simulink model "sampleModel106"  (R2022a)
settings: Solver=VariableStepAuto  StartTime=0.0  StopTime=10.0  RelTol=1e-3
undefined symbols (not defined in the file): DiscIntNeverNeededParam, magnitude, Newton, Raphson
libraries: simulink x379, slpidlib x89
(part 5 of 16)

== system sampleModel106/cfblk82/cfblk7/cfblk7 ==
  cfblk1 : Inport
  cfblk14 : Inport  Port=2
  cfblk15 : Inport  Port=3
  cfblk16 : Inport  Port=4
  cfblk10 : Constant  Value=[138530855.287176]  SampleTime=1
  cfblk11 : Constant  Value=[847049310.105778]  SampleTime=1
  cfblk12 : Subsystem
  cfblk13 : Subsystem
  cfblk17 : Delay  SampleTime=1
  cfblk18 : Delay  SampleTime=1
  cfblk3 : DiscreteFilter  SampleTime=1
  cfblk4 : simulink/Discrete/Transfer Fcn Real Zero  ZeroZ=0.75  ICPrevInput=0.0  DoSatur=off
      settings: SourceProductBaseCode=SL
  cfblk5 : DiscreteTransferFcn  SampleTime=1
  cfblk6 : DiscreteFilter  SampleTime=1
  cfblk7 : Sum  Inputs=+-
  cfblk8 : Assignment  DiagnosticForDimensions=Warning  IndexOptions=Index vector (dialog)  Indices=1  OutputSizes=1
  cfblk9 : Abs  SaturateOnIntegerOverflow=off
  cfblk2 : Outport
  wires:
  cfblk3/1 -> cfblk8/1, cfblk7/2
  cfblk10/1 -> cfblk12/1(cfblk1)
  cfblk9/1 -> cfblk13/1(cfblk1)
  cfblk15/1 -> cfblk12/2(cfblk6)
  cfblk11/1 -> cfblk2/1
  cfblk16/1 -> cfblk9/1
  cfblk6/1 -> cfblk4/1
  cfblk4/1 -> cfblk3/1
  cfblk8/1 -> cfblk5/1
  cfblk5/1 -> cfblk12/3(cfblk7)
  cfblk14/1 -> cfblk12/4(cfblk8)
  cfblk1/1 -> cfblk13/3(cfblk14)
  cfblk13/1(cfblk2) -> cfblk7/1
  cfblk13/2(cfblk15) -> cfblk6/1, cfblk12/5(cfblk9)
  cfblk7/1 -> cfblk17/1
  cfblk17/1 -> cfblk13/2(cfblk13)
  cfblk12/1(cfblk2) -> cfblk18/1
  cfblk18/1 -> cfblk8/2

== system sampleModel106/cfblk82/cfblk7/cfblk8 ==
  cfblk1 : Inport
  cfblk15 : Inport  Port=2
  cfblk10 : Constant  Value=[796043451.416910]  SampleTime=1
  cfblk11 : Subsystem
  cfblk12 : Subsystem
  cfblk13 : Subsystem
  cfblk14 : If  IfExpression=u1 >= 0  SampleTime=1
  cfblk18 : Subsystem  TreatAsAtomicUnit=on
  cfblk19 : Subsystem  TreatAsAtomicUnit=on
  cfblk20 : Delay  SampleTime=1
  cfblk21 : Delay  SampleTime=1
  cfblk22 : Delay  SampleTime=1
  cfblk3 : DiscreteZeroPole  Poles=[0 0.5]  Gain=1
  cfblk4 : DiscreteTransferFcn  SampleTime=1
  cfblk5 : Signum
  cfblk6 : Sum  Inputs=-+
  cfblk7 : UnaryMinus
  cfblk8 : Signum
  cfblk9 : UnaryMinus
  cfblk2 : Outport
  cfblk16 : Outport  Port=2
  cfblk17 : Outport  Port=3
  wires:
  cfblk19/1(cfblk2) -> cfblk12/2(cfblk6)
  cfblk15/1 -> cfblk14/1
  cfblk3/1 -> cfblk11/1(cfblk1)
  cfblk13/1(cfblk2) -> cfblk2/1
  cfblk12/1(cfblk2) -> cfblk8/1
  cfblk12/2(cfblk7) -> cfblk9/1
  cfblk4/1 -> cfblk5/1
  cfblk1/1 -> cfblk19/1(cfblk1)
  cfblk19/2(cfblk7) -> cfblk6/1
  cfblk6/1 -> cfblk3/1
  cfblk8/1 -> cfblk6/2
  cfblk18/1(cfblk2) -> cfblk16/1
  cfblk5/1 -> cfblk13/1(cfblk1)
  cfblk12/3(cfblk8) -> cfblk13/2(cfblk14)
  cfblk11/1(cfblk2) -> cfblk7/1
  cfblk18/2(cfblk7) -> cfblk4/1
  cfblk10/1 -> cfblk13/3(cfblk15)
  cfblk11/2(cfblk11) -> cfblk17/1
  cfblk11/3(cfblk12) -> cfblk13/4(cfblk16)
  cfblk14/1 -> cfblk18/Action
  cfblk14/2 -> cfblk19/Action
  cfblk7/1 -> cfblk20/1
  cfblk20/1 -> cfblk12/1(cfblk1)
  cfblk13/2(cfblk17) -> cfblk21/1
  cfblk21/1 -> cfblk11/2(cfblk10)
  cfblk9/1 -> cfblk22/1
  cfblk22/1 -> cfblk18/1(cfblk1)

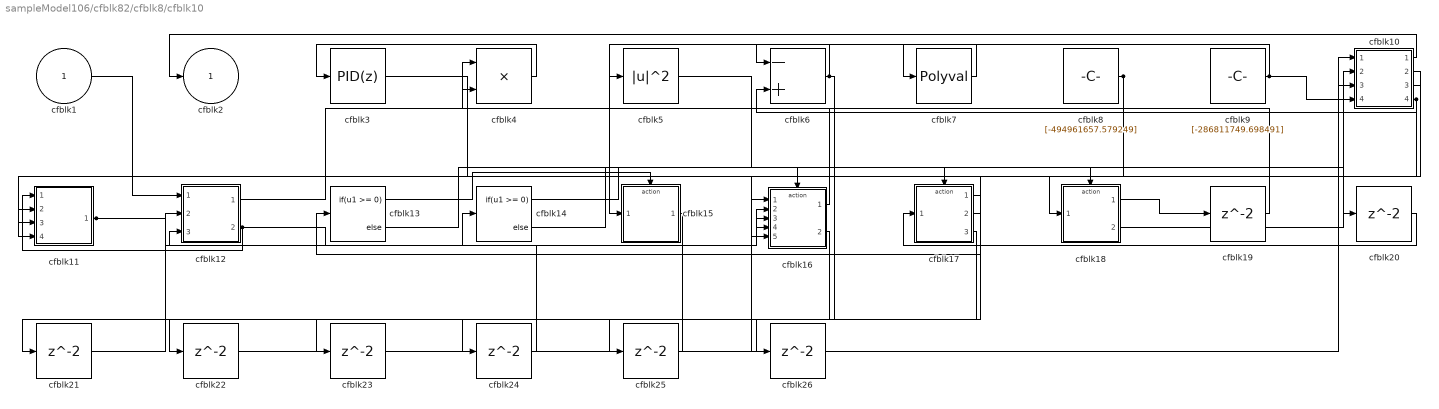
== system sampleModel106/cfblk82/cfblk8/cfblk10 ==
  cfblk1 : Inport
  cfblk10 : Subsystem
  cfblk11 : Subsystem
  cfblk12 : Subsystem
  cfblk13 : If  IfExpression=u1 >= 0  SampleTime=1
  cfblk14 : If  IfExpression=u1 >= 0  SampleTime=1
  cfblk15 : Subsystem  TreatAsAtomicUnit=on
  cfblk16 : Subsystem  TreatAsAtomicUnit=on
  cfblk17 : Subsystem  TreatAsAtomicUnit=on
  cfblk18 : Subsystem  TreatAsAtomicUnit=on
  cfblk{19..26} (8 alike) : Delay  SampleTime=1
  cfblk3 : slpidlib/PID Controller  Controller=PID  Form=Parallel  TimeDomain=Discrete-time  UseExternalTs=off  SampleTime=1  IntegratorMethod=Forward Euler  FilterMethod=Forward Euler  ControllerParametersSource=internal  P=1  I=1  UseKiTs=off  D=0  N=100  UseFilter=on  TunerSelectOption=Transfer Function Based (PID Tuner App)  InitialConditionSource=internal  InitialConditionForIntegrator=0  InitialConditionForFilter=0  DifferentiatorICPrevScaledInput=0  ExternalReset=none  TrackingMode=off  Kt=1  LimitOutput=off  SatLimitsSource=internal  UpperSaturationLimit=inf  LowerSaturationLimit=-inf  LinearizeAsGain=off  AntiWindupMode=none  Kb=1  POutMin=[]  POutMax=[]  IOutMin=[]  IOutMax=[]  DOutMin=[]  DOutMax=[]  NOutMin=[]  NOutMax=[]  SumOutMin=[]  SumOutMax=[]  SaturationOutMin=[]  SaturationOutMax=[]  PParamMin=[]  PParamMax=[]  IParamMin=[]  IParamMax=[]  DParamMin=[]  DParamMax=[]  NParamMin=[]  NParamMax=[]  KbParamMin=[]  KbParamMax=[]  KtParamMin=[]  KtParamMax=[]  KbOutMin=[]  KbOutMax=[]  KtOutMin=[]  KtOutMax=[]  IntegratorOutMin=[]  IntegratorOutMax=[]  FilterOutMin=[]  FilterOutMax=[]  SumI1OutMin=[]  SumI1OutMax=[]  SumI2OutMin=[]  SumI2OutMax=[]  SumI3OutMin=[]  SumI3OutMax=[]  SumI4OutMin=[]  SumI4OutMax=[]  SumDOutMin=[]  SumDOutMax=[]  DifferentiatorOutMin=[]  DifferentiatorOutMax=[]  FilterDiffOutCoefMin=[]  FilterDiffOutCoefMax=[]  ReciprocalOutMin=[]  ReciprocalOutMax=[]  SumDenOutMin=[]  SumDenOutMax=[]  SumNumOutMin=[]  SumNumOutMax=[]  DivideOutMin=[]  DivideOutMax=[]  UdiffTsProdOutMin=[]  UdiffTsProdOutMax=[]  NTsProdOutMin=[]  NTsProdOutMax=[]  UintegralTsProdOutMin=[]  UintegralTsProdOutMax=[]  UngainTsProdOutMin=[]  UngainTsProdOutMax=[]  IntegratorContinuousStateAttributes=''  IntegratorStateMustResolveToSignalObject=off  IntegratorRTWStateStorageClass=Auto  FilterContinuousStateAttributes=''  FilterStateMustResolveToSignalObject=off  FilterRTWStateStorageClass=Auto  ParallelPVariant=InternalParameters  IdealPVariant=Disabled  IVariant=InternalParameters  DVariant=InternalParameters  IntegratorVariant=Discrete  SatVariant=Disabled  AWVariant=Passthrough  PCopyVariant=Disabled  TRVariant=Disabled  FdbkBlocksVariant=Forward  IdealPFdbkVariant=Disabled  SatFdbkVariant=Disabled  DerivativeFilterVariant=ForwardEulerFilter  NVariant=InternalParameters  NCopyVariant=Disabled  FilterICVariant=InternalICsFilter  IntegratorICVariant=InternalICs  ExternalResetVariant=Disabled  TRSumVariant=Passthrough  SumFdbkVariant=Disabled  SumVariant=Sum_PID  TsampFilterVariant=InternalTs  TsampNgainVariant=Passthrough  TsampIntegralVariant=Passthrough  ExternalSaturationOutDataTypeStr=Inherit: Same as second input  aMode=0
  cfblk4 : Product
  cfblk5 : Math  Operator=magnitude^2
  cfblk6 : Sum  Inputs=-+
  cfblk7 : Polyval  Coefs=[ +2.081618890e-019, -1.441693666e-014, +4.719686976e-010, -8.536869453e-006, +1.621573104e-001, -8.087801117e+001 ]
  cfblk8 : Constant  Value=[-494961657.579249]  SampleTime=1
  cfblk9 : Constant  Value=[-286811749.698491]  SampleTime=1
  cfblk2 : Outport
  wires:
  cfblk1/1 -> cfblk12/1(cfblk1)
  cfblk9/1 -> cfblk7/1, cfblk10/4(cfblk12)
  cfblk8/1 -> cfblk13/1, cfblk16/5(cfblk15)
  cfblk4/1 -> cfblk3/1
  cfblk6/1 -> cfblk15/1(cfblk1), cfblk26/1
  cfblk7/1 -> cfblk6/1
  cfblk3/1 -> cfblk18/1(cfblk1)
  cfblk12/1(cfblk2) -> cfblk4/1
  cfblk12/2(cfblk11) -> cfblk11/1(cfblk1), cfblk16/4(cfblk14)
  cfblk10/1(cfblk2) -> cfblk2/1
  cfblk16/1(cfblk2) -> cfblk5/1
  cfblk11/1(cfblk2) -> cfblk16/2(cfblk12), cfblk16/3(cfblk13)
  cfblk10/2(cfblk13) -> cfblk11/2(cfblk11)
  cfblk18/2(cfblk13) -> cfblk10/2(cfblk10)
  cfblk10/3(cfblk14) -> cfblk11/3(cfblk12)
  cfblk10/4(cfblk15) -> cfblk6/2, cfblk11/4(cfblk13)
  cfblk13/1 -> cfblk15/Action
  cfblk13/2 -> cfblk16/Action
  cfblk14/1 -> cfblk17/Action
  cfblk14/2 -> cfblk18/Action
  cfblk18/1(cfblk2) -> cfblk19/1
  cfblk19/1 -> cfblk4/2
  cfblk5/1 -> cfblk20/1
  cfblk20/1 -> cfblk17/1(cfblk1)
  cfblk17/1(cfblk2) -> cfblk21/1
  cfblk21/1 -> cfblk12/2(cfblk9)
  cfblk17/2(cfblk10) -> cfblk22/1
  cfblk22/1 -> cfblk16/1(cfblk1)
  cfblk17/3(cfblk11) -> cfblk23/1
  cfblk23/1 -> cfblk10/1(cfblk1)
  cfblk16/2(cfblk16) -> cfblk24/1
  cfblk24/1 -> cfblk14/1
  cfblk15/1(cfblk2) -> cfblk25/1
  cfblk25/1 -> cfblk12/3(cfblk10)
  cfblk26/1 -> cfblk10/3(cfblk11)

== system sampleModel106/cfblk83/cfblk11/cfblk10 ==
  cfblk1 : Inport
  cfblk12 : Inport  Port=2
  cfblk10 : Constant  Value=[-915348538.475738]  SampleTime=1
  cfblk11 : If  IfExpression=u1 >= 0  SampleTime=1
  cfblk14 : Subsystem  TreatAsAtomicUnit=on
  cfblk15 : Subsystem  TreatAsAtomicUnit=on
  cfblk{16..20} (5 alike) : Delay  SampleTime=1
  cfblk3 : DiscreteIntegrator  ICPrevOutput=DiscIntNeverNeededParam  ICPrevScaledInput=DiscIntNeverNeededParam
  cfblk4 : simulink/Discrete/Transfer Fcn Lead or Lag  PoleZ=0.95  ZeroZ=0.75  ICPrevOutput=0.0  ICPrevInput=0.0  DoSatur=off
      settings: SourceProductBaseCode=SL
  cfblk5 : UnitDelay  HasFrameUpgradeWarning=on
  cfblk6 : Sum  Inputs=|++
  cfblk7 : Squeeze
  cfblk8 : Sum  Inputs=+-
  cfblk9 : Sum  Inputs=|++
  cfblk2 : Outport
  cfblk13 : Outport  Port=2
  wires:
  cfblk5/1 -> cfblk2/1, cfblk16/1
  cfblk3/1 -> cfblk7/1
  cfblk4/1 -> cfblk8/1
  cfblk12/1 -> cfblk14/1(cfblk1)
  cfblk14/1(cfblk2) -> cfblk15/2(cfblk13)
  cfblk9/1 -> cfblk4/1
  cfblk8/1 -> cfblk6/1, cfblk14/3(cfblk7)
  cfblk6/1 -> cfblk11/1
  cfblk15/1(cfblk2) -> cfblk5/1, cfblk3/1, cfblk18/1
  cfblk1/1 -> cfblk9/2
  cfblk10/1 -> cfblk14/2(cfblk6)
  cfblk14/3(cfblk10) -> cfblk13/1, cfblk15/3(cfblk14), cfblk20/1
  cfblk11/1 -> cfblk14/Action
  cfblk11/2 -> cfblk15/Action
  cfblk16/1 -> cfblk8/2
  cfblk7/1 -> cfblk17/1
  cfblk17/1 -> cfblk15/1(cfblk1)
  cfblk18/1 -> cfblk14/4(cfblk8)
  cfblk14/2(cfblk9) -> cfblk19/1
  cfblk19/1 -> cfblk9/1
  cfblk20/1 -> cfblk6/2

== system sampleModel106/cfblk83/cfblk11/cfblk11 ==
  cfblk1 : Inport
  cfblk6 : Inport  Port=2
  cfblk3 : DiscreteFir  SampleTime=1
  cfblk4 : simulink/Discrete/Difference  ICPrevInput=0.0  OutMin=[]  OutMax=[]  OutDataTypeStr=Inherit: Inherit via back propagation  OutDataType=fixdt(1, 16)  OutScaling=2^-10  DoSatur=off
  cfblk5 : Constant  Value=[980742649.522338]  SampleTime=1
  cfblk2 : Outport
  cfblk7 : Outport  Port=2
  cfblk8 : Outport  Port=3
  wires:
  cfblk1/1 -> cfblk7/1
  cfblk3/1 -> cfblk4/1
  cfblk4/1 -> cfblk8/1
  cfblk5/1 -> cfblk3/1
  cfblk6/1 -> cfblk2/1

== system sampleModel106/cfblk83/cfblk11/cfblk8 ==
  cfblk1 : Inport
  cfblk10 : Inport  Port=2
  cfblk11 : Delay  SampleTime=1
  cfblk3 : DiscreteIntegrator  ICPrevOutput=DiscIntNeverNeededParam  ICPrevScaledInput=DiscIntNeverNeededParam
  cfblk4 : Delay  DelayLengthSource=Input port  SampleTime=1
      settings: InputPortMap=u0,p1
  cfblk5 : Sqrt  Operator=rSqrt  AlgorithmType=Newton-Raphson
  cfblk6 : Abs  SaturateOnIntegerOverflow=off
  cfblk7 : DotProduct  OutDataTypeStr=Inherit: Inherit via internal rule
  cfblk8 : Constant  Value=[987587050.518951]  SampleTime=1
  cfblk9 : Subsystem
  cfblk2 : Outport
  wires:
  cfblk7/1 -> cfblk4/1
  cfblk10/1 -> cfblk5/1
  cfblk1/1 -> cfblk9/1(cfblk1)
  cfblk5/1 -> cfblk9/2(cfblk10)
  cfblk3/1 -> cfblk6/1
  cfblk6/1 -> cfblk7/2
  cfblk8/1 -> cfblk9/3(cfblk11)
  cfblk9/1(cfblk2) -> cfblk3/1
  cfblk9/2(cfblk12) -> cfblk2/1
  cfblk9/3(cfblk13) -> cfblk4/2
  cfblk4/1 -> cfblk11/1
  cfblk11/1 -> cfblk7/1

== system sampleModel106/cfblk83/cfblk11/cfblk9 ==
  cfblk1 : Inport
  cfblk10 : Inport  Port=2
  cfblk11 : Inport  Port=3
  cfblk14 : Delay  SampleTime=1
  cfblk3 : Sqrt  Operator=rSqrt  AlgorithmType=Newton-Raphson
  cfblk4 : Math  Operator=hypot
  cfblk5 : Constant  Value=[429893517.810689]  SampleTime=1
  cfblk6 : Constant  Value=[-633040645.705457]  SampleTime=1
  cfblk7 : Subsystem
  cfblk8 : Subsystem
  cfblk9 : Subsystem
  cfblk2 : Outport
  cfblk12 : Outport  Port=2
  cfblk13 : Outport  Port=3
  wires:
  cfblk9/1(cfblk2) -> cfblk7/1(cfblk1)
  cfblk8/1(cfblk2) -> cfblk7/2(cfblk10)
  cfblk6/1 -> cfblk8/1(cfblk1)
  cfblk11/1 -> cfblk13/1, cfblk9/3(cfblk16)
  cfblk8/2(cfblk8) -> cfblk2/1
  cfblk7/1(cfblk2) -> cfblk3/1
  cfblk10/1 -> cfblk12/1
  cfblk7/2(cfblk12) -> cfblk4/1
  cfblk1/1 -> cfblk9/1(cfblk1)
  cfblk5/1 -> cfblk9/2(cfblk15)
  cfblk3/1 -> cfblk4/2
  cfblk4/1 -> cfblk14/1
  cfblk14/1 -> cfblk7/3(cfblk11)

== system sampleModel106/cfblk83/cfblk12/cfblk11 ==
  cfblk1 : Inport
  cfblk6 : Inport  Port=2
  cfblk7 : Inport  Port=3
  cfblk8 : Inport  Port=4
  cfblk3 : Gain  Gain=[-783620375.475826]
  cfblk4 : Signum
  cfblk5 : Constant  Value=[572148918.887176]  SampleTime=1
  cfblk2 : Outport
  cfblk9 : Outport  Port=2
  wires:
  cfblk4/1 -> cfblk3/1
  cfblk3/1 -> cfblk2/1
  cfblk7/1 -> cfblk9/1
  cfblk8/1 -> cfblk4/1

== system sampleModel106/cfblk83/cfblk12/cfblk12 ==
  cfblk1 : Inport
  cfblk12 : Inport  Port=2
  cfblk10 : Subsystem
  cfblk11 : Subsystem
  cfblk{14..17} (4 alike) : Delay  SampleTime=1
  cfblk3 : Rounding
  cfblk4 : MinMax  Function=max  Inputs=3
  cfblk5 : Product  Inputs=**
  cfblk6 : MinMax  Function=max  Inputs=3
  cfblk7 : Sum  Inputs=+-
  cfblk8 : Constant  Value=[584813353.823935]  SampleTime=1
  cfblk9 : Constant  Value=[-958735761.055608]  SampleTime=1
  cfblk2 : Outport
  cfblk13 : Outport  Port=2
  wires:
  cfblk6/1 -> cfblk5/1, cfblk10/3(cfblk11)
  cfblk12/1 -> cfblk3/1, cfblk10/1(cfblk1), cfblk4/3
  cfblk5/1 -> cfblk11/1(cfblk1), cfblk10/2(cfblk10)
  cfblk8/1 -> cfblk4/1
  cfblk1/1 -> cfblk2/1
  cfblk11/1(cfblk2) -> cfblk7/1, cfblk4/2, cfblk10/4(cfblk12), cfblk10/5(cfblk13)
  cfblk9/1 -> cfblk6/2
  cfblk4/1 -> cfblk7/2
  cfblk3/1 -> cfblk6/3
  cfblk10/3(cfblk15) -> cfblk13/1, cfblk17/1
  cfblk7/1 -> cfblk14/1
  cfblk14/1 -> cfblk6/1
  cfblk10/1(cfblk2) -> cfblk15/1
  cfblk15/1 -> cfblk11/2(cfblk11)
  cfblk10/2(cfblk14) -> cfblk16/1
  cfblk16/1 -> cfblk5/2
  cfblk17/1 -> cfblk11/3(cfblk12)

== system sampleModel106/cfblk83/cfblk12/cfblk13 ==
  cfblk1 : Inport
  cfblk11 : Inport  Port=2
  cfblk10 : Subsystem
  cfblk13 : Delay  SampleTime=1
  cfblk3 : DiscreteStateSpace
  cfblk4 : Delay  SampleTime=1
  cfblk5 : UnitDelay  HasFrameUpgradeWarning=on
  cfblk6 : Sum  Inputs=+
  cfblk7 : Constant  Value=[139757462.378631]  SampleTime=1
  cfblk8 : Subsystem
  cfblk9 : Subsystem
  cfblk2 : Outport
  cfblk12 : Outport  Port=2
  wires:
  cfblk8/1(cfblk2) -> cfblk5/1
  cfblk7/1 -> cfblk4/1
  cfblk1/1 -> cfblk10/1(cfblk1)
  cfblk11/1 -> cfblk9/1(cfblk1)
  cfblk10/1(cfblk2) -> cfblk3/1
  cfblk8/2(cfblk15) -> cfblk9/2(cfblk13)
  cfblk9/1(cfblk2) -> cfblk12/1
  cfblk6/1 -> cfblk8/1(cfblk1)
  cfblk5/1 -> cfblk2/1
  cfblk4/1 -> cfblk6/1
  cfblk8/3(cfblk16) -> cfblk9/3(cfblk14)
  cfblk3/1 -> cfblk8/3(cfblk14)
  cfblk8/4(cfblk17) -> cfblk9/4(cfblk15)
  cfblk10/2(cfblk15) -> cfblk9/5(cfblk16)
  cfblk9/2(cfblk17) -> cfblk13/1
  cfblk13/1 -> cfblk8/2(cfblk13)

== system sampleModel106/cfblk83/cfblk13/cfblk11 ==
  cfblk1 : Inport
  cfblk10 : Inport  Port=2
  cfblk11 : Delay  SampleTime=1
  cfblk3 : DiscreteIntegrator  ICPrevOutput=DiscIntNeverNeededParam  ICPrevScaledInput=DiscIntNeverNeededParam
  cfblk4 : Sin  TimeSource=Use external signal  SampleTime=0
  cfblk5 : Product  Inputs=**
  cfblk6 : DotProduct  OutDataTypeStr=Inherit: Inherit via internal rule
  cfblk7 : Constant  Value=[480451020.421901]  SampleTime=1
  cfblk8 : Constant  Value=[724826496.666308]  SampleTime=1
  cfblk9 : Subsystem
  cfblk2 : Outport
  wires:
  cfblk3/1 -> cfblk5/1
  cfblk1/1 -> cfblk3/1
  cfblk6/1 -> cfblk4/1
  cfblk9/1(cfblk2) -> cfblk6/2
  cfblk7/1 -> cfblk2/1
  cfblk5/1 -> cfblk9/1(cfblk1)
  cfblk10/1 -> cfblk5/2
  cfblk8/1 -> cfblk9/2(cfblk12)
  cfblk4/1 -> cfblk11/1
  cfblk11/1 -> cfblk6/1

== system sampleModel106/cfblk83/cfblk13/cfblk12 ==
  cfblk1 : Inport
  cfblk{9..15} (7 alike) : Delay  SampleTime=1
  cfblk3 : MinMax  Inputs=2
  cfblk4 : Abs  SaturateOnIntegerOverflow=off
  cfblk5 : Subsystem
  cfblk6 : Subsystem
  cfblk7 : Subsystem
  cfblk8 : Subsystem
  cfblk2 : Outport
  wires:
  cfblk4/1 -> cfblk6/1(cfblk1), cfblk15/1
  cfblk6/1(cfblk2) -> cfblk7/1(cfblk1)
  cfblk3/1 -> cfblk7/4(cfblk14), cfblk13/1, cfblk14/1
  cfblk1/1 -> cfblk8/2(cfblk7), cfblk5/6(cfblk15), cfblk2/1
  cfblk6/2(cfblk14) -> cfblk7/2(cfblk12)
  cfblk5/1(cfblk2) -> cfblk4/1
  cfblk6/3(cfblk15) -> cfblk3/1, cfblk3/2, cfblk11/1, cfblk12/1
  cfblk8/1(cfblk2) -> cfblk5/4(cfblk13)
  cfblk5/2(cfblk17) -> cfblk7/3(cfblk13), cfblk7/5(cfblk15)
  cfblk7/1(cfblk2) -> cfblk9/1
  cfblk9/1 -> cfblk5/1(cfblk1)
  cfblk7/2(cfblk16) -> cfblk10/1
  cfblk10/1 -> cfblk5/2(cfblk11)
  cfblk11/1 -> cfblk5/3(cfblk12)
  cfblk12/1 -> cfblk8/3(cfblk8)
  cfblk13/1 -> cfblk8/1(cfblk1)
  cfblk14/1 -> cfblk5/7(cfblk16)
  cfblk15/1 -> cfblk5/5(cfblk14)

== system sampleModel106/cfblk83/cfblk13/cfblk13 ==
  cfblk1 : Inport
  cfblk10 : Inport  Port=2
  cfblk13 : Delay  SampleTime=1
  cfblk14 : Delay  SampleTime=1
  cfblk15 : Delay  SampleTime=1
  cfblk3 : DiscreteFilter  SampleTime=1
  cfblk4 : simulink/Discrete/Transfer Fcn Real Zero  ZeroZ=0.75  ICPrevInput=0.0  DoSatur=off
      settings: SourceProductBaseCode=SL
  cfblk5 : Sum  Inputs=+-
  cfblk6 : Rounding
  cfblk7 : Sum  Inputs=+
  cfblk8 : Subsystem
  cfblk9 : Subsystem
  cfblk2 : Outport
  cfblk11 : Outport  Port=2
  cfblk12 : Outport  Port=3
  wires:
  cfblk9/1(cfblk2) -> cfblk3/1
  cfblk9/2(cfblk12) -> cfblk11/1
  cfblk1/1 -> cfblk7/1, cfblk8/3(cfblk11)
  cfblk3/1 -> cfblk4/1
  cfblk4/1 -> cfblk5/1
  cfblk10/1 -> cfblk12/1, cfblk5/2
  cfblk7/1 -> cfblk2/1
  cfblk5/1 -> cfblk13/1, cfblk14/1
  cfblk8/1(cfblk2) -> cfblk9/1(cfblk1)
  cfblk8/2(cfblk12) -> cfblk6/1
  cfblk13/1 -> cfblk8/2(cfblk10)
  cfblk14/1 -> cfblk9/2(cfblk11)
  cfblk6/1 -> cfblk15/1
  cfblk15/1 -> cfblk8/1(cfblk1)

== system sampleModel106/cfblk84/cfblk10/cfblk10 ==
  cfblk1 : Inport
  cfblk12 : Inport  Port=2
  cfblk13 : Inport  Port=3
  cfblk14 : Inport  Port=4
  cfblk10 : Subsystem
  cfblk11 : Subsystem
  cfblk17 : Delay
  cfblk3 : Sum  Inputs=|++
  cfblk4 : Product
  cfblk5 : Sin  TimeSource=Use external signal  SampleTime=0
  cfblk6 : Gain  Gain=[836498416.139520]
  cfblk7 : Constant  Value=[-865016845.781020]  SampleTime=1
  cfblk8 : Constant  Value=[-866150485.828076]  SampleTime=1
  cfblk9 : Constant  Value=[-175857800.113051]  SampleTime=1
  cfblk2 : Outport
  cfblk15 : Outport  Port=2
  cfblk16 : Outport  Port=3
  wires:
  cfblk13/1 -> cfblk2/1
  cfblk8/1 -> cfblk10/1(cfblk1)
  cfblk4/1 -> cfblk6/1
  cfblk1/1 -> cfblk5/1
  cfblk9/1 -> cfblk4/1
  cfblk12/1 -> cfblk4/2
  cfblk11/1(cfblk2) -> cfblk10/2(cfblk6)
  cfblk7/1 -> cfblk3/1
  cfblk5/1 -> cfblk11/2(cfblk7)
  cfblk14/1 -> cfblk15/1
  cfblk6/1 -> cfblk3/2
  cfblk10/2(cfblk7) -> cfblk16/1
  cfblk10/1(cfblk2) -> cfblk17/1
  cfblk17/1 -> cfblk11/1(cfblk1)

== system sampleModel106/cfblk84/cfblk10/cfblk8 ==
  cfblk1 : Inport
  cfblk9 : Inport  Port=2
  cfblk10 : Inport  Port=3
  cfblk11 : Inport  Port=4
  cfblk12 : Inport  Port=5
  cfblk13 : DataTypeConversion  SaturateOnIntegerOverflow=off  RndMeth=Floor
  cfblk3 : DiscreteFir
  cfblk4 : UnaryMinus
  cfblk5 : PermuteDimensions
  cfblk6 : Constant  Value=[-987508818.835473]  SampleTime=1
  cfblk7 : Constant  Value=[432958284.413679]  SampleTime=1
  cfblk8 : Subsystem
  cfblk2 : Outport
  wires:
  cfblk6/1 -> cfblk5/1
  cfblk11/1 -> cfblk3/1
  cfblk10/1 -> cfblk2/1
  cfblk3/1 -> cfblk8/1(cfblk1)
  cfblk1/1 -> cfblk13/1
  cfblk13/1 -> cfblk4/1

== system sampleModel106/cfblk84/cfblk10/cfblk9 ==
  cfblk1 : Inport
  cfblk7 : Inport  Port=2
  cfblk8 : Inport  Port=3
  cfblk12 : Delay
  cfblk3 : Constant  Value=[860292327.118658]  SampleTime=1
  cfblk4 : Constant  Value=[-448193708.153886]  SampleTime=1
  cfblk5 : Subsystem
  cfblk6 : Subsystem
  cfblk2 : Outport
  cfblk9 : Outport  Port=2
  cfblk10 : Outport  Port=3
  cfblk11 : Outport  Port=4
  wires:
  cfblk3/1 -> cfblk6/1(cfblk1), cfblk6/5(cfblk12)
  cfblk6/1(cfblk2) -> cfblk9/1, cfblk12/1
  cfblk4/1 -> cfblk5/1(cfblk1), cfblk6/4(cfblk11)
  cfblk7/1 -> cfblk2/1
  cfblk8/1 -> cfblk10/1
  cfblk1/1 -> cfblk5/2(cfblk6), cfblk11/1, cfblk6/3(cfblk10)
  cfblk5/1(cfblk2) -> cfblk6/2(cfblk9)
  cfblk12/1 -> cfblk5/3(cfblk7)

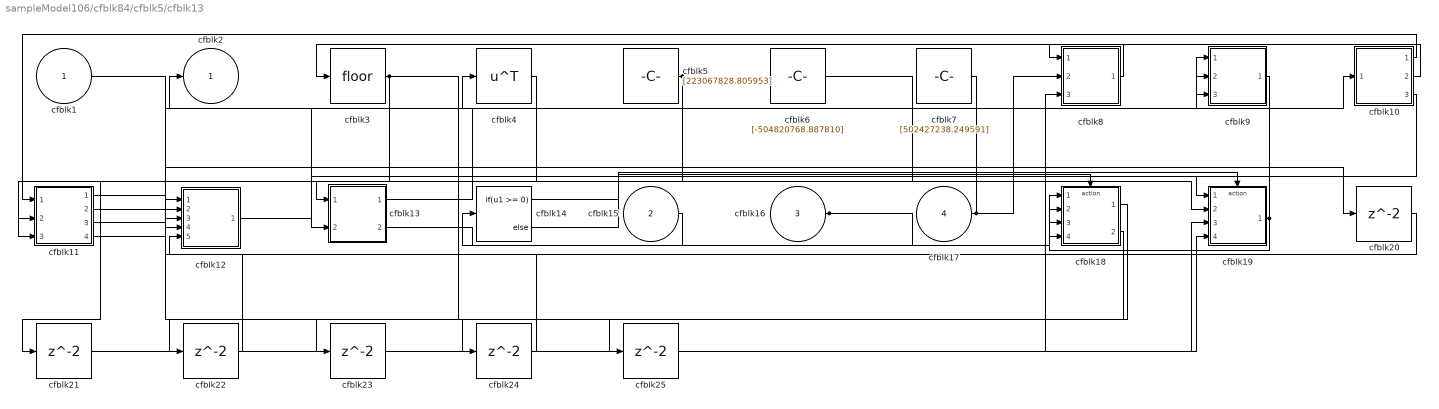
== system sampleModel106/cfblk84/cfblk5/cfblk13 ==
  cfblk1 : Inport
  cfblk15 : Inport  Port=2
  cfblk16 : Inport  Port=3
  cfblk17 : Inport  Port=4
  cfblk10 : Subsystem
  cfblk11 : Subsystem
  cfblk12 : Subsystem
  cfblk13 : Subsystem
  cfblk14 : If  IfExpression=u1 >= 0  SampleTime=1
  cfblk18 : Subsystem  TreatAsAtomicUnit=on
  cfblk19 : Subsystem  TreatAsAtomicUnit=on
  cfblk{20..25} (6 alike) : Delay  SampleTime=1
  cfblk3 : Rounding
  cfblk4 : Math  Operator=transpose
  cfblk5 : Constant  Value=[223067828.805953]  SampleTime=1
  cfblk6 : Constant  Value=[-504820768.887810]  SampleTime=1
  cfblk7 : Constant  Value=[502427238.249591]  SampleTime=1
  cfblk8 : Subsystem
  cfblk9 : Subsystem
  cfblk2 : Outport
  wires:
  cfblk17/1 -> cfblk2/1, cfblk8/2(cfblk16)
  cfblk8/1(cfblk2) -> cfblk3/1
  cfblk3/1 -> cfblk13/1(cfblk1), cfblk25/1
  cfblk10/1(cfblk2) -> cfblk11/1(cfblk1)
  cfblk1/1 -> cfblk12/2(cfblk11)
  cfblk16/1 -> cfblk18/1(cfblk1), cfblk18/3(cfblk15)
  cfblk7/1 -> cfblk12/3(cfblk12)
  cfblk12/1(cfblk2) -> cfblk10/1(cfblk1)
  cfblk9/1(cfblk2) -> cfblk19/1(cfblk1)
  cfblk19/1(cfblk2) -> cfblk4/1, cfblk18/4(cfblk16)
  cfblk5/1 -> cfblk11/2(cfblk7), cfblk11/3(cfblk8)
  cfblk10/2(cfblk12) -> cfblk8/1(cfblk1)
  cfblk6/1 -> cfblk19/2(cfblk11)
  cfblk15/1 -> cfblk14/1
  cfblk11/2(cfblk9) -> cfblk9/1(cfblk1)
  cfblk10/3(cfblk13) -> cfblk13/2(cfblk9)
  cfblk13/1(cfblk2) -> cfblk9/2(cfblk11)
  cfblk11/4(cfblk11) -> cfblk9/3(cfblk12)
  cfblk13/2(cfblk10) -> cfblk18/2(cfblk14)
  cfblk14/1 -> cfblk18/Action
  cfblk14/2 -> cfblk19/Action
  cfblk11/1(cfblk2) -> cfblk20/1
  cfblk20/1 -> cfblk12/4(cfblk13)
  cfblk4/1 -> cfblk21/1
  cfblk21/1 -> cfblk19/4(cfblk13)
  cfblk18/1(cfblk2) -> cfblk22/1
  cfblk22/1 -> cfblk12/1(cfblk1)
  cfblk18/2(cfblk17) -> cfblk23/1
  cfblk23/1 -> cfblk19/3(cfblk12)
  cfblk11/3(cfblk10) -> cfblk24/1
  cfblk24/1 -> cfblk12/5(cfblk14)
  cfblk25/1 -> cfblk8/3(cfblk17)

== system sampleModel106/cfblk84/cfblk5/cfblk14 ==
  cfblk1 : Inport
  cfblk10 : Gain  Gain=[-554957442.246404]
  cfblk11 : Constant  Value=[-424613233.201941]  SampleTime=1
  cfblk12 : Constant  Value=[487603603.932364]  SampleTime=1
  cfblk13 : Constant  Value=[-769270987.130435]  SampleTime=1
  cfblk15 : Delay  SampleTime=1
  cfblk3 : slpidlib/PID Controller (2DOF)  Controller=PID  Form=Parallel  TimeDomain=Discrete-time  UseExternalTs=off  SampleTime=1  IntegratorMethod=Forward Euler  FilterMethod=Forward Euler  ControllerParametersSource=internal  P=1  I=1  UseKiTs=off  D=0  N=100  UseFilter=on  b=1  c=1  TunerSelectOption=Transfer Function Based (PID Tuner App)  InitialConditionSource=internal  InitialConditionForIntegrator=0  InitialConditionForFilter=0  DifferentiatorICPrevScaledInput=0  ExternalReset=none  TrackingMode=off  Kt=1  LimitOutput=off  SatLimitsSource=internal  UpperSaturationLimit=inf  LowerSaturationLimit=-inf  LinearizeAsGain=off  AntiWindupMode=none  Kb=1  POutMin=[]  POutMax=[]  IOutMin=[]  IOutMax=[]  DOutMin=[]  DOutMax=[]  NOutMin=[]  NOutMax=[]  bOutMin=[]  bOutMax=[]  cOutMin=[]  cOutMax=[]  SumOutMin=[]  SumOutMax=[]  SaturationOutMin=[]  SaturationOutMax=[]  PParamMin=[]  PParamMax=[]  IParamMin=[]  IParamMax=[]  DParamMin=[]  DParamMax=[]  NParamMin=[]  NParamMax=[]  bParamMin=[]  bParamMax=[]  cParamMin=[]  cParamMax=[]  KbParamMin=[]  KbParamMax=[]  KtParamMin=[]  KtParamMax=[]  KbOutMin=[]  KbOutMax=[]  KtOutMin=[]  KtOutMax=[]  IntegratorOutMin=[]  IntegratorOutMax=[]  FilterOutMin=[]  FilterOutMax=[]  SumI1OutMin=[]  SumI1OutMax=[]  SumI2OutMin=[]  SumI2OutMax=[]  SumI3OutMin=[]  SumI3OutMax=[]  SumI4OutMin=[]  SumI4OutMax=[]  SumDOutMin=[]  SumDOutMax=[]  Sum1OutMin=[]  Sum1OutMax=[]  Sum2OutMin=[]  Sum2OutMax=[]  Sum3OutMin=[]  Sum3OutMax=[]  DifferentiatorOutMin=[]  DifferentiatorOutMax=[]  FilterDiffOutCoefMin=[]  FilterDiffOutCoefMax=[]  ReciprocalOutMin=[]  ReciprocalOutMax=[]  SumDenOutMin=[]  SumDenOutMax=[]  SumNumOutMin=[]  SumNumOutMax=[]  DivideOutMin=[]  DivideOutMax=[]  UdiffTsProdOutMin=[]  UdiffTsProdOutMax=[]  NTsProdOutMin=[]  NTsProdOutMax=[]  UintegralTsProdOutMin=[]  UintegralTsProdOutMax=[]  UngainTsProdOutMin=[]  UngainTsProdOutMax=[]  IntegratorContinuousStateAttributes=''  IntegratorStateMustResolveToSignalObject=off  IntegratorRTWStateStorageClass=Auto  FilterContinuousStateAttributes=''  FilterStateMustResolveToSignalObject=off  FilterRTWStateStorageClass=Auto  ParallelPVariant=InternalParameters  IdealPVariant=Disabled  IVariant=InternalParameters  DVariant=InternalParameters  bVariant=InternalParameters  cVariant=InternalParameters  IntegratorVariant=Discrete  SatVariant=Disabled  AWVariant=Passthrough  PCopyVariant=Disabled  TRVariant=Disabled  FdbkBlocksVariant=Forward  IdealPFdbkVariant=Disabled  SatFdbkVariant=Disabled  DerivativeFilterVariant=ForwardEulerFilter  NVariant=InternalParameters  NCopyVariant=Disabled  FilterICVariant=InternalICsFilter  IntegratorICVariant=InternalICs  ExternalResetVariant=Disabled  TRSumVariant=Passthrough  SumFdbkVariant=Disabled  SumVariant=Sum_PID  TsampFilterVariant=InternalTs  TsampNgainVariant=Passthrough  TsampIntegralVariant=Passthrough  ExternalSaturationOutDataTypeStr=Inherit: Same as second input
      settings: SourceProductBaseCode=SL
  cfblk4 : Sum  Inputs=+-
  cfblk5 : Sum  Inputs=+
  cfblk6 : Rounding
  cfblk7 : Product  Inputs=*
  cfblk8 : Sqrt  Operator=rSqrt  AlgorithmType=Newton-Raphson
  cfblk9 : Sin  TimeSource=Use external signal  SampleTime=0
  cfblk2 : Outport
  cfblk14 : Outport  Port=2
  wires:
  cfblk12/1 -> cfblk6/1
  cfblk10/1 -> cfblk2/1
  cfblk13/1 -> cfblk9/1
  cfblk11/1 -> cfblk10/1
  cfblk5/1 -> cfblk3/1
  cfblk7/1 -> cfblk14/1
  cfblk1/1 -> cfblk7/1
  cfblk6/1 -> cfblk8/1
  cfblk9/1 -> cfblk5/1
  cfblk3/1 -> cfblk4/1
  cfblk8/1 -> cfblk4/2
  cfblk4/1 -> cfblk15/1
  cfblk15/1 -> cfblk3/2

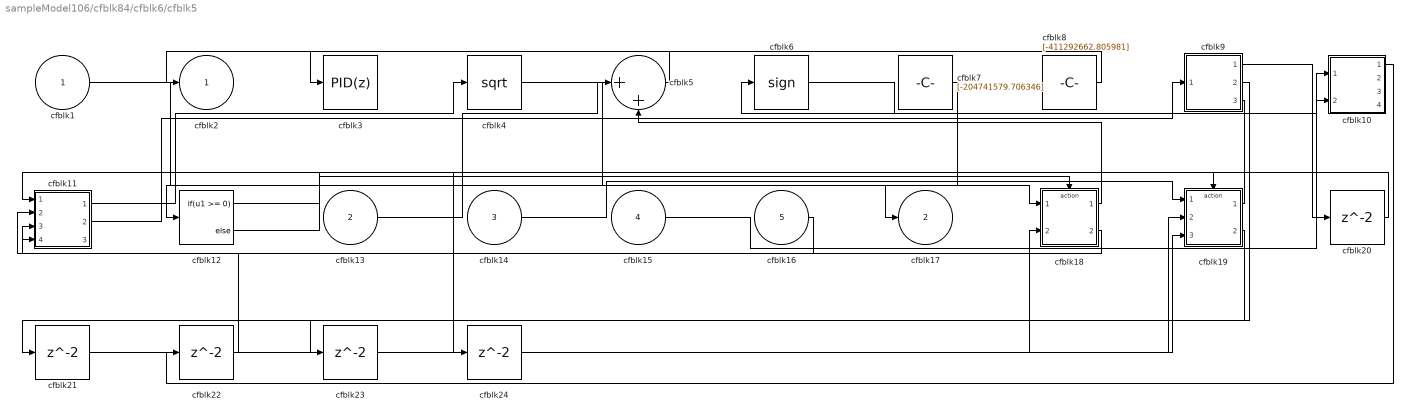
== system sampleModel106/cfblk84/cfblk6/cfblk5 ==
  cfblk1 : Inport
  cfblk13 : Inport  Port=2
  cfblk14 : Inport  Port=3
  cfblk15 : Inport  Port=4
  cfblk16 : Inport  Port=5
  cfblk10 : Subsystem
  cfblk11 : Subsystem
  cfblk12 : If  IfExpression=u1 >= 0  SampleTime=1
  cfblk18 : Subsystem  TreatAsAtomicUnit=on
  cfblk19 : Subsystem  TreatAsAtomicUnit=on
  cfblk{20..24} (5 alike) : Delay  SampleTime=1
  cfblk3 : slpidlib/PID Controller  Controller=PID  Form=Parallel  TimeDomain=Discrete-time  UseExternalTs=off  SampleTime=1  IntegratorMethod=Forward Euler  FilterMethod=Forward Euler  ControllerParametersSource=internal  P=1  I=1  UseKiTs=off  D=0  N=100  UseFilter=on  TunerSelectOption=Transfer Function Based (PID Tuner App)  InitialConditionSource=internal  InitialConditionForIntegrator=0  InitialConditionForFilter=0  DifferentiatorICPrevScaledInput=0  ExternalReset=none  TrackingMode=off  Kt=1  LimitOutput=off  SatLimitsSource=internal  UpperSaturationLimit=inf  LowerSaturationLimit=-inf  LinearizeAsGain=off  AntiWindupMode=none  Kb=1  POutMin=[]  POutMax=[]  IOutMin=[]  IOutMax=[]  DOutMin=[]  DOutMax=[]  NOutMin=[]  NOutMax=[]  SumOutMin=[]  SumOutMax=[]  SaturationOutMin=[]  SaturationOutMax=[]  PParamMin=[]  PParamMax=[]  IParamMin=[]  IParamMax=[]  DParamMin=[]  DParamMax=[]  NParamMin=[]  NParamMax=[]  KbParamMin=[]  KbParamMax=[]  KtParamMin=[]  KtParamMax=[]  KbOutMin=[]  KbOutMax=[]  KtOutMin=[]  KtOutMax=[]  IntegratorOutMin=[]  IntegratorOutMax=[]  FilterOutMin=[]  FilterOutMax=[]  SumI1OutMin=[]  SumI1OutMax=[]  SumI2OutMin=[]  SumI2OutMax=[]  SumI3OutMin=[]  SumI3OutMax=[]  SumI4OutMin=[]  SumI4OutMax=[]  SumDOutMin=[]  SumDOutMax=[]  DifferentiatorOutMin=[]  DifferentiatorOutMax=[]  FilterDiffOutCoefMin=[]  FilterDiffOutCoefMax=[]  ReciprocalOutMin=[]  ReciprocalOutMax=[]  SumDenOutMin=[]  SumDenOutMax=[]  SumNumOutMin=[]  SumNumOutMax=[]  DivideOutMin=[]  DivideOutMax=[]  UdiffTsProdOutMin=[]  UdiffTsProdOutMax=[]  NTsProdOutMin=[]  NTsProdOutMax=[]  UintegralTsProdOutMin=[]  UintegralTsProdOutMax=[]  UngainTsProdOutMin=[]  UngainTsProdOutMax=[]  IntegratorContinuousStateAttributes=''  IntegratorStateMustResolveToSignalObject=off  IntegratorRTWStateStorageClass=Auto  FilterContinuousStateAttributes=''  FilterStateMustResolveToSignalObject=off  FilterRTWStateStorageClass=Auto  ParallelPVariant=InternalParameters  IdealPVariant=Disabled  IVariant=InternalParameters  DVariant=InternalParameters  IntegratorVariant=Discrete  SatVariant=Disabled  AWVariant=Passthrough  PCopyVariant=Disabled  TRVariant=Disabled  FdbkBlocksVariant=Forward  IdealPFdbkVariant=Disabled  SatFdbkVariant=Disabled  DerivativeFilterVariant=ForwardEulerFilter  NVariant=InternalParameters  NCopyVariant=Disabled  FilterICVariant=InternalICsFilter  IntegratorICVariant=InternalICs  ExternalResetVariant=Disabled  TRSumVariant=Passthrough  SumFdbkVariant=Disabled  SumVariant=Sum_PID  TsampFilterVariant=InternalTs  TsampNgainVariant=Passthrough  TsampIntegralVariant=Passthrough  ExternalSaturationOutDataTypeStr=Inherit: Same as second input  aMode=0
  cfblk4 : Sqrt
  cfblk5 : Sum  Inputs=|++
  cfblk6 : Signum
  cfblk7 : Constant  Value=[-204741579.706346]  SampleTime=1
  cfblk8 : Constant  Value=[-411292662.805981]  SampleTime=1
  cfblk9 : Subsystem
  cfblk2 : Outport
  cfblk17 : Outport  Port=2
  wires:
  cfblk8/1 -> cfblk3/1
  cfblk7/1 -> cfblk12/1
  cfblk11/1(cfblk2) -> cfblk4/1
  cfblk15/1 -> cfblk10/1(cfblk1)
  cfblk4/1 -> cfblk17/1
  cfblk1/1 -> cfblk18/1(cfblk1)
  cfblk13/1 -> cfblk5/1
  cfblk14/1 -> cfblk19/1(cfblk1)
  cfblk19/1(cfblk2) -> cfblk6/1
  cfblk5/1 -> cfblk2/1
  cfblk11/2(cfblk15) -> cfblk9/1(cfblk1)
  cfblk6/1 -> cfblk10/2(cfblk12)
  cfblk18/1(cfblk2) -> cfblk5/2
  cfblk18/2(cfblk9) -> cfblk11/3(cfblk13)
  cfblk16/1 -> cfblk11/4(cfblk14)
  cfblk12/1 -> cfblk18/Action
  cfblk12/2 -> cfblk19/Action
  cfblk9/1(cfblk2) -> cfblk20/1
  cfblk20/1 -> cfblk11/1(cfblk1)
  cfblk9/2(cfblk6) -> cfblk21/1
  cfblk21/1 -> cfblk19/2(cfblk6)
  cfblk10/1(cfblk2) -> cfblk22/1
  cfblk22/1 -> cfblk11/2(cfblk12)
  cfblk19/2(cfblk8) -> cfblk23/1
  cfblk23/1 -> cfblk18/2(cfblk8)
  cfblk9/3(cfblk7) -> cfblk24/1
  cfblk24/1 -> cfblk19/3(cfblk7)

== system sampleModel106/cfblk84/cfblk6/cfblk6 ==
  cfblk1 : Inport
  cfblk10 : Subsystem
  cfblk11 : Subsystem
  cfblk12 : Subsystem
  cfblk13 : Subsystem
  cfblk{15..19} (5 alike) : Delay  SampleTime=1
  cfblk3 : Delay  ShowEnablePort=on  SampleTime=1
      settings: InputPortMap=u0,e6
  cfblk4 : Rounding
  cfblk5 : Product
  cfblk6 : Sum  Inputs=|++
  cfblk7 : Constant  Value=[-151219371.354714]  SampleTime=1
  cfblk8 : Constant  Value=[776463646.241198]  SampleTime=1
  cfblk9 : Constant  Value=[-351809939.384547]  SampleTime=1
  cfblk2 : Outport
  cfblk14 : Outport  Port=2
  wires:
  cfblk4/1 -> cfblk11/1(cfblk1)
  cfblk10/1(cfblk2) -> cfblk14/1
  cfblk1/1 -> cfblk10/1(cfblk1), cfblk13/5(cfblk7)
  cfblk8/1 -> cfblk10/2(cfblk13)
  cfblk5/1 -> cfblk3/1
  cfblk13/1(cfblk2) -> cfblk3/2
  cfblk6/1 -> cfblk4/1
  cfblk12/2(cfblk10) -> cfblk13/1(cfblk1)
  cfblk12/3(cfblk11) -> cfblk13/2(cfblk4)
  cfblk13/3(cfblk9) -> cfblk5/1
  cfblk9/1 -> cfblk5/2
  cfblk11/3(cfblk7) -> cfblk2/1, cfblk12/2(cfblk8)
  cfblk7/1 -> cfblk13/4(cfblk6), cfblk6/2, cfblk12/3(cfblk9)
  cfblk10/2(cfblk17) -> cfblk6/1
  cfblk11/1(cfblk2) -> cfblk15/1
  cfblk15/1 -> cfblk10/3(cfblk14)
  cfblk11/2(cfblk6) -> cfblk16/1
  cfblk16/1 -> cfblk10/4(cfblk15)
  cfblk12/1(cfblk2) -> cfblk17/1
  cfblk17/1 -> cfblk10/5(cfblk16)
  cfblk3/1 -> cfblk18/1
  cfblk18/1 -> cfblk13/3(cfblk5)
  cfblk13/2(cfblk8) -> cfblk19/1
  cfblk19/1 -> cfblk12/1(cfblk1)

== system sampleModel106/cfblk84/cfblk6/cfblk7 ==
  cfblk1 : Inport
  cfblk12 : Inport  Port=2
  cfblk10 : Subsystem
  cfblk11 : If  IfExpression=u1 >= 0  SampleTime=1
  cfblk13 : Subsystem  TreatAsAtomicUnit=on
  cfblk14 : Subsystem  TreatAsAtomicUnit=on
  cfblk{15..23} (9 alike) : Delay  SampleTime=1
  cfblk3 : Bias  Bias=[185659872.506394]  SaturateOnIntegerOverflow=off
  cfblk4 : Constant  Value=[378728154.377516]  SampleTime=1
  cfblk5 : Subsystem
  cfblk6 : Subsystem
  cfblk7 : Subsystem
  cfblk8 : Subsystem
  cfblk9 : Subsystem
  cfblk2 : Outport
  wires:
  cfblk4/1 -> cfblk8/1(cfblk1)
  cfblk1/1 -> cfblk10/1(cfblk1)
  cfblk9/1(cfblk2) -> cfblk11/1
  cfblk13/1(cfblk2) -> cfblk3/1
  cfblk10/1(cfblk2) -> cfblk2/1
  cfblk14/1(cfblk2) -> cfblk6/3(cfblk16), cfblk21/1
  cfblk10/2(cfblk15) -> cfblk9/1(cfblk1)
  cfblk13/2(cfblk12) -> cfblk8/2(cfblk8)
  cfblk13/3(cfblk13) -> cfblk5/1(cfblk1)
  cfblk12/1 -> cfblk13/5(cfblk11), cfblk7/5(cfblk10)
  cfblk9/2(cfblk6) -> cfblk5/2(cfblk10)
  cfblk8/1(cfblk2) -> cfblk7/1(cfblk1)
  cfblk7/3(cfblk12) -> cfblk6/1(cfblk1)
  cfblk10/3(cfblk16) -> cfblk9/4(cfblk5)
  cfblk10/4(cfblk17) -> cfblk7/2(cfblk7), cfblk6/2(cfblk15)
  cfblk9/3(cfblk7) -> cfblk7/3(cfblk8)
  cfblk9/4(cfblk8) -> cfblk7/4(cfblk9)
  cfblk11/1 -> cfblk13/Action
  cfblk11/2 -> cfblk14/Action
  cfblk3/1 -> cfblk15/1
  cfblk15/1 -> cfblk13/3(cfblk9)
  cfblk7/1(cfblk2) -> cfblk16/1
  cfblk16/1 -> cfblk13/4(cfblk10)
  cfblk7/2(cfblk11) -> cfblk17/1
  cfblk17/1 -> cfblk9/3(cfblk4)
  cfblk6/1(cfblk2) -> cfblk18/1
  cfblk18/1 -> cfblk10/2(cfblk14)
  cfblk6/2(cfblk17) -> cfblk19/1
  cfblk19/1 -> cfblk8/3(cfblk9)
  cfblk5/1(cfblk2) -> cfblk20/1
  cfblk20/1 -> cfblk14/1(cfblk1)
  cfblk21/1 -> cfblk13/1(cfblk1)
  cfblk5/2(cfblk11) -> cfblk22/1
  cfblk22/1 -> cfblk13/2(cfblk8)
  cfblk5/3(cfblk12) -> cfblk23/1
  cfblk23/1 -> cfblk9/2(cfblk3)

== system sampleModel106/cfblk84/cfblk9/cfblk10 ==
  cfblk1 : Inport
  cfblk11 : Inport  Port=2
  cfblk10 : If  IfExpression=u1 >= 0  SampleTime=1
  cfblk12 : Subsystem  TreatAsAtomicUnit=on
  cfblk13 : Subsystem  TreatAsAtomicUnit=on
  cfblk{14..21} (8 alike) : Delay
  cfblk3 : Delay  DelayLengthSource=Input port
      settings: InputPortMap=u0,p1
  cfblk4 : Gain  Gain=[-229166448.360161]
  cfblk5 : Product  Inputs=**
  cfblk6 : Trigonometry
  cfblk7 : Subsystem
  cfblk8 : Subsystem
  cfblk9 : Subsystem
  cfblk2 : Outport
  wires:
  cfblk11/1 -> cfblk12/1(cfblk1)
  cfblk4/1 -> cfblk3/1, cfblk18/1
  cfblk8/1(cfblk2) -> cfblk4/1
  cfblk13/1(cfblk2) -> cfblk5/1
  cfblk12/1(cfblk2) -> cfblk3/2
  cfblk1/1 -> cfblk2/1, cfblk13/3(cfblk14)
  cfblk6/1 -> cfblk7/3(cfblk10), cfblk14/1
  cfblk8/2(cfblk10) -> cfblk19/1, cfblk20/1
  cfblk9/1(cfblk2) -> cfblk6/1
  cfblk13/2(cfblk15) -> cfblk9/2(cfblk5)
  cfblk5/1 -> cfblk9/3(cfblk6)
  cfblk9/2(cfblk7) -> cfblk8/1(cfblk1)
  cfblk13/3(cfblk16) -> cfblk7/1(cfblk1)
  cfblk7/2(cfblk11) -> cfblk8/2(cfblk8)
  cfblk13/4(cfblk17) -> cfblk7/2(cfblk9), cfblk12/5(cfblk16)
  cfblk7/4(cfblk13) -> cfblk8/3(cfblk9)
  cfblk10/1 -> cfblk12/Action
  cfblk10/2 -> cfblk13/Action
  cfblk14/1 -> cfblk9/1(cfblk1)
  cfblk7/1(cfblk2) -> cfblk15/1
  cfblk15/1 -> cfblk12/2(cfblk13)
  cfblk3/1 -> cfblk16/1
  cfblk16/1 -> cfblk10/1
  cfblk12/2(cfblk17) -> cfblk17/1
  cfblk17/1 -> cfblk5/2
  cfblk18/1 -> cfblk12/4(cfblk15)
  cfblk19/1 -> cfblk12/3(cfblk14)
  cfblk20/1 -> cfblk13/2(cfblk13)
  cfblk7/3(cfblk12) -> cfblk21/1
  cfblk21/1 -> cfblk13/1(cfblk1)

== system sampleModel106/cfblk84/cfblk9/cfblk11 ==
  cfblk1 : Inport
  cfblk13 : Inport  Port=2
  cfblk10 : Subsystem
  cfblk11 : Subsystem
  cfblk12 : Subsystem
  cfblk{4,16..19} (5 alike) : Delay
  cfblk3 : simulink/Discrete/Transfer Fcn Lead or Lag  PoleZ=0.95  ZeroZ=0.75  ICPrevOutput=0.0  ICPrevInput=0.0  DoSatur=off
      settings: SourceProductBaseCode=SL
  cfblk5 : Gain  Gain=[27160301.981311]
  cfblk6 : Gain  Gain=[-798340712.621102]
  cfblk7 : Assignment  DiagnosticForDimensions=Warning  IndexOptions=Index vector (dialog)  Indices=1  OutputSizes=1
  cfblk8 : Sum  Inputs=+-
  cfblk9 : Subsystem
  cfblk2 : Outport
  cfblk14 : Outport  Port=2
  cfblk15 : Outport  Port=3
  wires:
  cfblk6/1 -> cfblk11/1(cfblk1)
  cfblk10/1(cfblk2) -> cfblk15/1, cfblk7/2
  cfblk7/1 -> cfblk9/1(cfblk1)
  cfblk3/1 -> cfblk4/1
  cfblk9/1(cfblk2) -> cfblk8/1
  cfblk11/1(cfblk2) -> cfblk8/2
  cfblk11/2(cfblk7) -> cfblk2/1
  cfblk12/1(cfblk2) -> cfblk5/1
  cfblk5/1 -> cfblk3/1, cfblk17/1
  cfblk8/1 -> cfblk12/2(cfblk6)
  cfblk13/1 -> cfblk6/1
  cfblk1/1 -> cfblk10/2(cfblk15)
  cfblk12/2(cfblk8) -> cfblk14/1, cfblk18/1
  cfblk4/1 -> cfblk16/1
  cfblk16/1 -> cfblk12/1(cfblk1)
  cfblk17/1 -> cfblk12/3(cfblk7)
  cfblk18/1 -> cfblk7/1
  cfblk9/2(cfblk7) -> cfblk19/1
  cfblk19/1 -> cfblk10/1(cfblk1)

== system sampleModel106/cfblk84/cfblk9/cfblk12 ==
  cfblk1 : Inport
  cfblk7 : Inport  Port=2
  cfblk3 : UnitDelay  SampleTime=-1  HasFrameUpgradeWarning=on
  cfblk4 : MinMax  Function=max
  cfblk5 : Subsystem
  cfblk6 : Subsystem
  cfblk8 : Delay
  cfblk9 : Delay
  cfblk2 : Outport
  wires:
  cfblk1/1 -> cfblk5/1(cfblk1)
  cfblk7/1 -> cfblk4/1
  cfblk6/1(cfblk2) -> cfblk2/1
  cfblk4/1 -> cfblk5/2(cfblk10)
  cfblk5/1(cfblk2) -> cfblk6/2(cfblk12)
  cfblk6/3(cfblk15) -> cfblk3/1
  cfblk5/2(cfblk12) -> cfblk6/3(cfblk13)
  cfblk6/2(cfblk14) -> cfblk8/1
  cfblk8/1 -> cfblk5/3(cfblk11)
  cfblk3/1 -> cfblk9/1
  cfblk9/1 -> cfblk6/1(cfblk1)

== system sampleModel106/cfblk84/cfblk9/cfblk13 ==
  cfblk1 : Inport
  cfblk12 : Inport  Port=2
  cfblk13 : Inport  Port=3
  cfblk10 : Subsystem
  cfblk11 : Subsystem
  cfblk15 : Delay
  cfblk16 : Delay
  cfblk3 : simulink/Discrete/Transfer Fcn Real Zero  ZeroZ=0.75  ICPrevInput=0.0  DoSatur=off
      settings: SourceProductBaseCode=SL
  cfblk4 : Sin  TimeSource=Use external signal  SampleTime=0
  cfblk5 : ComplexToRealImag
  cfblk6 : Product
  cfblk7 : Constant  Value=[239924137.082466]  SampleTime=1
  cfblk8 : Subsystem
  cfblk9 : Subsystem
  cfblk2 : Outport
  cfblk14 : Outport  Port=2
  wires:
  cfblk1/1 -> cfblk10/1(cfblk1)
  cfblk10/1(cfblk2) -> cfblk2/1
  cfblk12/1 -> cfblk5/1
  cfblk13/1 -> cfblk6/1
  cfblk8/2(cfblk11) -> cfblk4/1
  cfblk3/1 -> cfblk6/2
  cfblk5/1 -> cfblk9/1(cfblk1)
  cfblk5/2 -> cfblk11/2(cfblk5)
  cfblk8/3(cfblk12) -> cfblk14/1
  cfblk6/1 -> cfblk11/3(cfblk6)
  cfblk7/1 -> cfblk9/2(cfblk12)
  cfblk9/1(cfblk2) -> cfblk8/1(cfblk1)
  cfblk9/2(cfblk13) -> cfblk8/2(cfblk9)
  cfblk11/1(cfblk2) -> cfblk8/3(cfblk10)
  cfblk8/1(cfblk2) -> cfblk15/1
  cfblk15/1 -> cfblk3/1
  cfblk4/1 -> cfblk16/1
  cfblk16/1 -> cfblk11/1(cfblk1)

== system sampleModel106/cfblk86/cfblk10/cfblk10 ==
  cfblk1 : Inport
  cfblk7 : Inport  Port=2
  cfblk3 : Sum  Inputs=|++
  cfblk4 : Constant  Value=[-952140755.794251]  SampleTime=1
  cfblk5 : Subsystem
  cfblk6 : Subsystem
  cfblk8 : Delay
  cfblk2 : Outport
  wires:
  cfblk1/1 -> cfblk2/1, cfblk5/3(cfblk9), cfblk5/4(cfblk10)
  cfblk6/1(cfblk2) -> cfblk3/1
  cfblk7/1 -> cfblk5/1(cfblk1)
  cfblk5/1(cfblk2) -> cfblk6/1(cfblk1)
  cfblk4/1 -> cfblk3/2, cfblk5/5(cfblk11)
  cfblk5/2(cfblk12) -> cfblk6/2(cfblk8)
  cfblk3/1 -> cfblk8/1
  cfblk8/1 -> cfblk5/2(cfblk8)

== system sampleModel106/cfblk86/cfblk10/cfblk11 ==
  cfblk1 : Inport
  cfblk10 : Inport  Port=2
  cfblk11 : Inport  Port=3
  cfblk3 : DiscreteFilter
  cfblk4 : Sin  TimeSource=Use external signal  SampleTime=0
  cfblk5 : Sqrt
  cfblk6 : Constant  Value=[186701262.844114]  SampleTime=1
  cfblk7 : Constant  Value=[-865714998.881079]  SampleTime=1
  cfblk8 : Constant  Value=[801557178.258104]  SampleTime=1
  cfblk9 : Subsystem
  cfblk2 : Outport
  cfblk12 : Outport  Port=2
  wires:
  cfblk10/1 -> cfblk4/1
  cfblk5/1 -> cfblk12/1
  cfblk11/1 -> cfblk2/1
  cfblk8/1 -> cfblk9/1(cfblk1)
  cfblk9/1(cfblk2) -> cfblk3/1
  cfblk1/1 -> cfblk5/1

== system sampleModel106/cfblk86/cfblk10/cfblk12 ==
  cfblk1 : Inport
  cfblk7 : Inport  Port=2
  cfblk8 : Inport  Port=3
  cfblk9 : Inport  Port=4
  cfblk11 : Delay
  cfblk3 : DiscreteIntegrator  SampleTime=-1  ICPrevOutput=DiscIntNeverNeededParam  ICPrevScaledInput=DiscIntNeverNeededParam
  cfblk4 : DotProduct  OutDataTypeStr=Inherit: Inherit via internal rule
  cfblk5 : simulink/Math Operations/Slider Gain  gain=1  low=0  high=2
  cfblk6 : Subsystem
  cfblk2 : Outport
  cfblk10 : Outport  Port=2
  wires:
  cfblk7/1 -> cfblk3/1
  cfblk8/1 -> cfblk10/1, cfblk2/1, cfblk6/4(cfblk11)
  cfblk1/1 -> cfblk5/1
  cfblk3/1 -> cfblk4/1
  cfblk9/1 -> cfblk6/1(cfblk1)
  cfblk5/1 -> cfblk6/3(cfblk10)
  cfblk6/1(cfblk2) -> cfblk4/2
  cfblk4/1 -> cfblk11/1
  cfblk11/1 -> cfblk6/2(cfblk9)

== system sampleModel106/cfblk86/cfblk10/cfblk13 ==
  cfblk1 : Inport
  cfblk12 : Inport  Port=2
  cfblk13 : Inport  Port=3
  cfblk10 : UnaryMinus
  cfblk11 : Subsystem
  cfblk15 : Delay
  cfblk3 : simulink/Discrete/Transfer Fcn First Order  PoleZ=0.95  ICPrevOutput=0.0  DoSatur=off
  cfblk4 : DiscreteFir
  cfblk5 : DiscreteZeroPole  Poles=[0 0.5]  Gain=1  SampleTime=-1
  cfblk6 : Squeeze
  cfblk7 : Rounding
  cfblk8 : Signum
  cfblk9 : PermuteDimensions
  cfblk2 : Outport
  cfblk14 : Outport  Port=2
  wires:
  cfblk3/1 -> cfblk6/1
  cfblk1/1 -> cfblk5/1
  cfblk6/1 -> cfblk9/1
  cfblk13/1 -> cfblk11/1(cfblk1)
  cfblk11/1(cfblk2) -> cfblk8/1
  cfblk7/1 -> cfblk10/1
  cfblk12/1 -> cfblk2/1
  cfblk5/1 -> cfblk4/1
  cfblk11/2(cfblk8) -> cfblk14/1
  cfblk8/1 -> cfblk7/1
  cfblk9/1 -> cfblk15/1
  cfblk15/1 -> cfblk3/1

== system sampleModel106/cfblk86/cfblk10/cfblk9 ==
  cfblk1 : Inport
  cfblk10 : Inport  Port=2
  cfblk11 : Delay
  cfblk3 : DiscreteStateSpace  SampleTime=-1
  cfblk4 : DiscreteFir
  cfblk5 : Product  Inputs=**
  cfblk6 : ComplexToMagnitudeAngle
  cfblk7 : Constant  Value=[-152285791.422154]  SampleTime=1
  cfblk8 : Subsystem
  cfblk9 : Subsystem
  cfblk2 : Outport
  wires:
  cfblk10/1 -> cfblk3/1
  cfblk8/1(cfblk2) -> cfblk2/1
  cfblk1/1 -> cfblk8/1(cfblk1)
  cfblk4/1 -> cfblk8/2(cfblk14)
  cfblk7/1 -> cfblk9/1(cfblk1)
  cfblk9/1(cfblk2) -> cfblk4/1
  cfblk5/1 -> cfblk6/1
  cfblk6/1 -> cfblk8/3(cfblk15)
  cfblk3/1 -> cfblk5/1
  cfblk6/2 -> cfblk11/1
  cfblk11/1 -> cfblk5/2

== system sampleModel106/cfblk86/cfblk11/cfblk7 ==
  cfblk1 : Inport
  cfblk12 : Subsystem  TreatAsAtomicUnit=on
  cfblk13 : Subsystem  TreatAsAtomicUnit=on
  cfblk{14..21} (8 alike) : Delay
  cfblk3 : Assignment  DiagnosticForDimensions=Warning  IndexOptions=Index vector (dialog)  Indices=1  OutputSizes=1
  cfblk4 : Sqrt  Operator=rSqrt  AlgorithmType=Newton-Raphson
  cfblk5 : Subsystem
  cfblk6 : Subsystem
  cfblk7 : Subsystem
  cfblk8 : Subsystem
  cfblk9 : If  IfExpression=u1 >= 0  SampleTime=1
  cfblk2 : Outport
  cfblk10 : Outport  Port=2
  cfblk11 : Outport  Port=3
  wires:
  cfblk13/1(cfblk2) -> cfblk17/1, cfblk18/1
  cfblk6/1(cfblk2) -> cfblk3/1
  cfblk8/1(cfblk2) -> cfblk12/2(cfblk12)
  cfblk12/2(cfblk14) -> cfblk4/1
  cfblk4/1 -> cfblk3/2, cfblk5/3(cfblk12)
  cfblk1/1 -> cfblk7/3(cfblk14), cfblk11/1
  cfblk12/3(cfblk15) -> cfblk13/1(cfblk1), cfblk6/2(cfblk7)
  cfblk5/2(cfblk13) -> cfblk6/1(cfblk1)
  cfblk7/1(cfblk2) -> cfblk8/2(cfblk16), cfblk13/3(cfblk13), cfblk5/2(cfblk11)
  cfblk5/3(cfblk14) -> cfblk10/1
  cfblk5/5(cfblk16) -> cfblk2/1
  cfblk9/1 -> cfblk12/Action
  cfblk9/2 -> cfblk13/Action
  cfblk12/1(cfblk2) -> cfblk14/1
  cfblk14/1 -> cfblk7/2(cfblk13)
  cfblk3/1 -> cfblk15/1
  cfblk15/1 -> cfblk7/1(cfblk1)
  cfblk5/1(cfblk2) -> cfblk16/1
  cfblk16/1 -> cfblk9/1
  cfblk17/1 -> cfblk12/1(cfblk1)
  cfblk18/1 -> cfblk5/1(cfblk1)
  cfblk6/2(cfblk8) -> cfblk19/1
  cfblk19/1 -> cfblk8/1(cfblk1)
  cfblk5/4(cfblk15) -> cfblk20/1
  cfblk20/1 -> cfblk13/2(cfblk12)
  cfblk5/6(cfblk17) -> cfblk21/1
  cfblk21/1 -> cfblk12/3(cfblk13)

== system sampleModel106/cfblk86/cfblk11/cfblk8 ==
  cfblk1 : Inport
  cfblk13 : Inport  Port=2
  cfblk14 : Inport  Port=3
  cfblk10 : Constant  Value=[-37205242.927428]  SampleTime=1
  cfblk11 : Subsystem
  cfblk12 : Subsystem
  cfblk16 : Delay
  cfblk17 : Delay
  cfblk3 : DiscreteTransferFcn
  cfblk4 : UnitDelay  SampleTime=-1  HasFrameUpgradeWarning=on
  cfblk5 : simulink/Discrete/Tapped Delay  vinit=0.0  samptime=-1  NumDelays=1  DelayOrder=Oldest  includeCurrent=off
  cfblk6 : Rounding
  cfblk7 : Signum
  cfblk8 : Assignment  DiagnosticForDimensions=Warning  IndexOptions=Index vector (dialog)  Indices=1  OutputSizes=1
  cfblk9 : Constant  Value=[514402338.401624]  SampleTime=1
  cfblk2 : Outport
  cfblk15 : Outport  Port=2
  wires:
  cfblk10/1 -> cfblk6/1
  cfblk14/1 -> cfblk2/1
  cfblk3/1 -> cfblk11/1(cfblk1)
  cfblk5/1 -> cfblk12/1(cfblk1)
  cfblk12/1(cfblk2) -> cfblk7/1
  cfblk1/1 -> cfblk11/2(cfblk7)
  cfblk11/1(cfblk2) -> cfblk15/1
  cfblk4/1 -> cfblk8/1
  cfblk9/1 -> cfblk12/2(cfblk9)
  cfblk13/1 -> cfblk3/1
  cfblk6/1 -> cfblk8/2
  cfblk8/1 -> cfblk16/1
  cfblk16/1 -> cfblk4/1
  cfblk7/1 -> cfblk17/1
  cfblk17/1 -> cfblk5/1

== system sampleModel106/cfblk86/cfblk12/cfblk10 ==
  cfblk1 : Inport
  cfblk10 : Rounding
  cfblk11 : Trigonometry
  cfblk12 : MinMax  Function=max  Inputs=2
  cfblk13 : Sin  TimeSource=Use external signal  SampleTime=0
  cfblk14 : Sqrt  Operator=rSqrt  AlgorithmType=Newton-Raphson
  cfblk15 : If  IfExpression=u1 >= 0  SampleTime=1
  cfblk17 : Subsystem  TreatAsAtomicUnit=on
  cfblk18 : Subsystem  TreatAsAtomicUnit=on
  cfblk{5,19..23} (6 alike) : Delay
  cfblk3 : simulink/Discrete/Tapped Delay  vinit=0.0  samptime=-1  NumDelays=1  DelayOrder=Oldest  includeCurrent=off
  cfblk4 : Delay  ShowEnablePort=on
      settings: InputPortMap=u0,e6
  cfblk6 : ComplexToMagnitudeAngle
  cfblk7 : Sum  Inputs=|++
  cfblk8 : Math  Operator=mod
  cfblk9 : Sum  Inputs=+-
  cfblk2 : Outport
  cfblk16 : Outport  Port=2
  wires:
  cfblk3/1 -> cfblk17/1(cfblk1), cfblk12/2
  cfblk13/1 -> cfblk18/1(cfblk1), cfblk12/1, cfblk5/1
  cfblk7/1 -> cfblk2/1, cfblk22/1
  cfblk10/1 -> cfblk9/1
  cfblk6/1 -> cfblk13/1
  cfblk4/1 -> cfblk11/1
  cfblk5/1 -> cfblk4/1, cfblk7/2
  cfblk17/1(cfblk2) -> cfblk8/2
  cfblk17/2(cfblk15) -> cfblk4/2
  cfblk18/2(cfblk12) -> cfblk9/2, cfblk7/1
  cfblk8/1 -> cfblk10/1
  cfblk6/2 -> cfblk14/1
  cfblk12/1 -> cfblk16/1
  cfblk1/1 -> cfblk17/2(cfblk14), cfblk3/1
  cfblk15/1 -> cfblk17/Action
  cfblk15/2 -> cfblk18/Action
  cfblk9/1 -> cfblk19/1
  cfblk19/1 -> cfblk8/1
  cfblk11/1 -> cfblk20/1
  cfblk20/1 -> cfblk18/2(cfblk10)
  cfblk18/1(cfblk2) -> cfblk21/1
  cfblk21/1 -> cfblk15/1
  cfblk22/1 -> cfblk18/3(cfblk11)
  cfblk14/1 -> cfblk23/1
  cfblk23/1 -> cfblk6/1

== system sampleModel106/cfblk86/cfblk12/cfblk11 ==
  cfblk1 : Inport
  cfblk13 : Inport  Port=2
  cfblk14 : Inport  Port=3
  cfblk10 : Subsystem
  cfblk11 : Subsystem
  cfblk12 : Subsystem
  cfblk3 : simulink/Discrete/Difference  ICPrevInput=0.0  OutMin=[]  OutMax=[]  OutDataTypeStr=Inherit: Inherit via back propagation  OutDataType=fixdt(1, 16)  OutScaling=2^-10  DoSatur=off
  cfblk4 : ComplexToMagnitudeAngle
  cfblk5 : simulink/Math Operations/Slider Gain  gain=1  low=0  high=2
  cfblk6 : Bias  Bias=[257366144.232323]  SaturateOnIntegerOverflow=off
  cfblk7 : Sum  Inputs=-+
  cfblk8 : Constant  Value=[-650429201.242789]  SampleTime=1
  cfblk9 : Constant  Value=[250175980.750585]  SampleTime=1
  cfblk2 : Outport
  wires:
  cfblk9/1 -> cfblk6/1
  cfblk6/1 -> cfblk3/1
  cfblk7/1 -> cfblk11/1(cfblk1)
  cfblk3/1 -> cfblk7/1
  cfblk13/1 -> cfblk4/1
  cfblk4/1 -> cfblk12/1(cfblk1)
  cfblk5/1 -> cfblk10/1(cfblk1)
  cfblk11/1(cfblk2) -> cfblk2/1
  cfblk14/1 -> cfblk11/2(cfblk10)
  cfblk8/1 -> cfblk7/2
  cfblk11/2(cfblk11) -> cfblk10/2(cfblk11)
  cfblk11/3(cfblk12) -> cfblk12/2(cfblk13)
  cfblk1/1 -> cfblk12/3(cfblk14)
  cfblk12/1(cfblk2) -> cfblk5/1
  cfblk12/2(cfblk15) -> cfblk10/3(cfblk12)
  cfblk4/2 -> cfblk10/4(cfblk13)
  cfblk11/4(cfblk13) -> cfblk10/5(cfblk14)
